simulink model "Speed_Limit_Adaptation"  (R2022b)
settings: configuration reference "CommonModelConfiguration" (kept outside this file)
undefined symbols (not defined in the file): cc_param_149, cc_param_23, cc_param_311, cc_param_36, LCFG_DSF_Timeout, LCFG_SetSpeedMinKPH_A3, LCFG_SetSpeedMinMPH_A3, LCFG_SLA_SetSpeedMaxKPH, LCFG_SLA_SetSpeedMaxMPH, LCFG_SLA_Timeout, LCFG_VehicleBrand
settings Model: Creator=RPETE142  LastModifiedBy=OTHOMSO1
settings ConfigSetRef: SourceName=CommonModelConfiguration  SourceLocation=Base Workspace

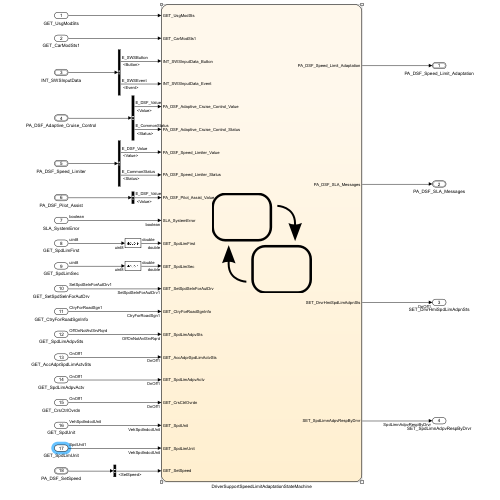
[thumbnail: Simulink's stored preview of the top-level diagram]
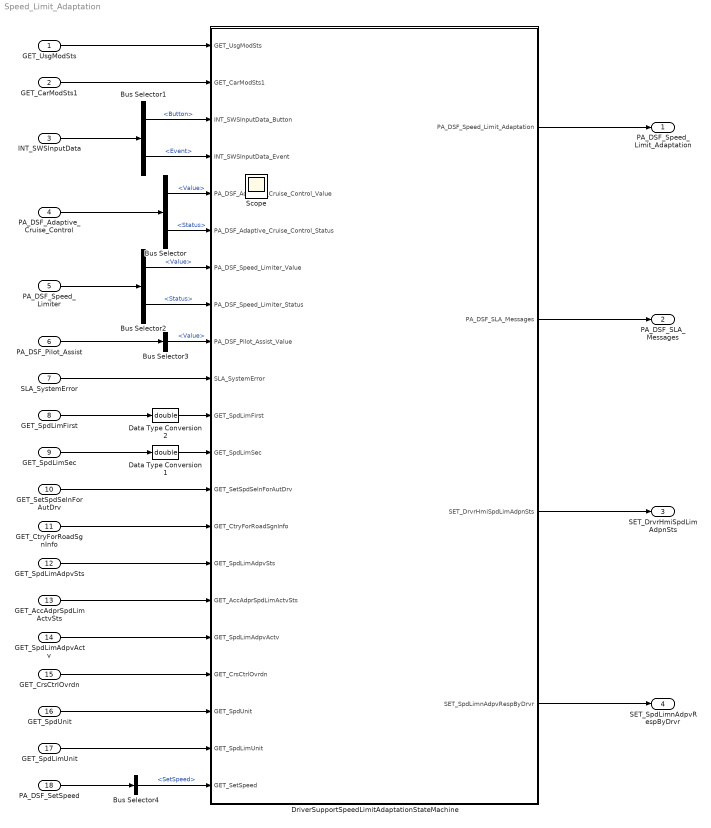
== system Speed_Limit_Adaptation ==
  GET_UsgModSts : Inport  SampleTime=0.01
  GET_CarModSts1 : Inport  Port=2
  INT_SWSInputData : Inport  Port=3  OutDataTypeStr=Bus: SWSInputData  LockScale=on
  PA_DSF_Adaptive_Cruise_Control : Inport  Port=4  OutDataTypeStr=Bus: PA_DSF_ACC
  PA_DSF_Speed_Limiter : Inport  Port=5  OutDataTypeStr=Bus: PA_DSF
  PA_DSF_Pilot_Assist : Inport  Port=6  OutDataTypeStr=Bus: PA_DSF
  SLA_SystemError : Inport  Port=7  OutDataTypeStr=boolean
  GET_SpdLimFirst : Inport  Port=8  OutDataTypeStr=SpdLimVal1
  GET_SpdLimSec : Inport  Port=9  OutDataTypeStr=SpdLimVal1
  GET_SetSpdSelnForAutDrv : Inport  Port=10  OutDataTypeStr=Enum: SetSpdSelnForAutDrv1
  GET_CtryForRoadSgnInfo : Inport  Port=11  OutDataTypeStr=Enum: CtryForRoadSgn1
  GET_SpdLimAdpvSts : Inport  Port=12  OutDataTypeStr=Enum: OffOnNotAvlSrvRqrd
  GET_AccAdprSpdLimActvSts : Inport  Port=13  OutDataTypeStr=Enum: OnOff1
  GET_SpdLimAdpvActv : Inport  Port=14  OutDataTypeStr=Enum: OnOff1
  GET_CrsCtrlOvrdn : Inport  Port=15  OutDataTypeStr=Enum: OnOff1
  GET_SpdUnit : Inport  Port=16  OutDataTypeStr=Enum: VehSpdIndcdUnit
  GET_SpdLimUnit : Inport  Port=17  OutDataTypeStr=Enum: SpdUnit1
  PA_DSF_SetSpeed : Inport  Port=18  OutDataTypeStr=Bus: PA_StatusAndValueAndDoubleAndDouble
  Bus Selector : BusSelector  OutputSignals=Value,Status
  Bus Selector1 : BusSelector  OutputSignals=Button,Event
  Bus Selector2 : BusSelector  OutputSignals=Value,Status
  Bus Selector3 : BusSelector  OutputSignals=Value
  Bus Selector4 : BusSelector  OutputSignals=SetSpeed
  Data Type Conversion1 : DataTypeConversion  OutDataTypeStr=double  SaturateOnIntegerOverflow=off  RndMeth=Floor  LockScale=on
  Data Type Conversion2 : DataTypeConversion  OutDataTypeStr=double  SaturateOnIntegerOverflow=off  RndMeth=Floor  LockScale=on
  "DriverSupportSpeedLimitAdaptationStateMachine " : Stateflow chart  TreatAsAtomicUnit=on
  PA_DSF_Speed_Limit_Adaptation : Outport  OutDataTypeStr=Bus: PA_DSF_SLA  VectorParamsAs1DForOutWhenUnconnected=off
  PA_DSF_SLA_Messages : Outport  Port=2  OutDataTypeStr=Bus: PA_DSF_Message  VectorParamsAs1DForOutWhenUnconnected=off
  SET_DrvrHmiSpdLimAdpnSts : Outport  Port=3  OutDataTypeStr=Enum: OnOff1  VectorParamsAs1DForOutWhenUnconnected=off
  SET_SpdLimnAdpvRespByDrvr : Outport  Port=4  OutDataTypeStr=Enum: SpdLimnAdpvRespByDrvr  VectorParamsAs1DForOutWhenUnconnected=off
  Scope : Scope
  wires:
  GET_UsgModSts/1 -> "DriverSupportSpeedLimitAdaptationStateMachine "/1(GET_UsgModSts)
  GET_CarModSts1/1 -> "DriverSupportSpeedLimitAdaptationStateMachine "/2(GET_CarModSts1)
  INT_SWSInputData/1 -> Bus Selector1/1
  Bus Selector1/2 -> "DriverSupportSpeedLimitAdaptationStateMachine "/4(INT_SWSInputData_Event)  "<Event>"
  Bus Selector1/1 -> "DriverSupportSpeedLimitAdaptationStateMachine "/3(INT_SWSInputData_Button)  "<Button>"
  Bus Selector/1 -> "DriverSupportSpeedLimitAdaptationStateMachine "/5(PA_DSF_Adaptive_Cruise_Control_Value)  "<Value>"
  PA_DSF_Adaptive_Cruise_Control/1 -> Bus Selector/1
  PA_DSF_Speed_Limiter/1 -> Bus Selector2/1
  PA_DSF_Pilot_Assist/1 -> Bus Selector3/1
  SLA_SystemError/1 -> "DriverSupportSpeedLimitAdaptationStateMachine "/10(SLA_SystemError)
  "DriverSupportSpeedLimitAdaptationStateMachine "/1(PA_DSF_Speed_Limit_Adaptation) -> PA_DSF_Speed_Limit_Adaptation/1
  GET_SpdLimFirst/1 -> Data Type Conversion2/1
  Data Type Conversion2/1 -> "DriverSupportSpeedLimitAdaptationStateMachine "/11(GET_SpdLimFirst)
  GET_SpdLimSec/1 -> Data Type Conversion1/1
  Data Type Conversion1/1 -> "DriverSupportSpeedLimitAdaptationStateMachine "/12(GET_SpdLimSec)
  GET_SetSpdSelnForAutDrv/1 -> "DriverSupportSpeedLimitAdaptationStateMachine "/13(GET_SetSpdSelnForAutDrv)
  GET_CtryForRoadSgnInfo/1 -> "DriverSupportSpeedLimitAdaptationStateMachine "/14(GET_CtryForRoadSgnInfo)
  Bus Selector/2 -> "DriverSupportSpeedLimitAdaptationStateMachine "/6(PA_DSF_Adaptive_Cruise_Control_Status)  "<Status>"
  Bus Selector2/1 -> "DriverSupportSpeedLimitAdaptationStateMachine "/7(PA_DSF_Speed_Limiter_Value)  "<Value>"
  Bus Selector2/2 -> "DriverSupportSpeedLimitAdaptationStateMachine "/8(PA_DSF_Speed_Limiter_Status)  "<Status>"
  Bus Selector3/1 -> "DriverSupportSpeedLimitAdaptationStateMachine "/9(PA_DSF_Pilot_Assist_Value)  "<Value>"
  "DriverSupportSpeedLimitAdaptationStateMachine "/3(SET_DrvrHmiSpdLimAdpnSts) -> SET_DrvrHmiSpdLimAdpnSts/1
  "DriverSupportSpeedLimitAdaptationStateMachine "/2(PA_DSF_SLA_Messages) -> PA_DSF_SLA_Messages/1
  GET_SpdLimAdpvSts/1 -> "DriverSupportSpeedLimitAdaptationStateMachine "/15(GET_SpdLimAdpvSts)
  GET_AccAdprSpdLimActvSts/1 -> "DriverSupportSpeedLimitAdaptationStateMachine "/16(GET_AccAdprSpdLimActvSts)
  GET_SpdLimAdpvActv/1 -> "DriverSupportSpeedLimitAdaptationStateMachine "/17(GET_SpdLimAdpvActv)
  "DriverSupportSpeedLimitAdaptationStateMachine "/4(SET_SpdLimnAdpvRespByDrvr) -> SET_SpdLimnAdpvRespByDrvr/1
  GET_CrsCtrlOvrdn/1 -> "DriverSupportSpeedLimitAdaptationStateMachine "/18(GET_CrsCtrlOvrdn)
  GET_SpdUnit/1 -> "DriverSupportSpeedLimitAdaptationStateMachine "/19(GET_SpdUnit)
  PA_DSF_SetSpeed/1 -> Bus Selector4/1
  Bus Selector4/1 -> "DriverSupportSpeedLimitAdaptationStateMachine "/21(GET_SetSpeed)  "<SetSpeed>"
  GET_SpdLimUnit/1 -> "DriverSupportSpeedLimitAdaptationStateMachine "/20(GET_SpdLimUnit)

== stateflow chart Speed_Limit_Adaptation/DriverSupportSpeedLimitAdaptationStateMachine  ==
  state CARCONFIG_INVALID
    entry:
    PA_DSF_Speed_Limit_Adaptation.Status = E_CommonStatus.NotPresent;
    PA_DSF_Speed_Limit_Adaptation.Value = E_DSF_Value.DSF_Off;
    PA_DSF_Speed_Limit_Adaptation.Format = false;
    PA_DSF_Speed_Limit_Adaptation.Data = 0;
    PA_DSF_SLA_Messages.Status = E_CommonStatus.NotPresent;
    PA_DSF_SLA_Messages.Value = E_DSF_Messages.Messages_Off;
    SET_DrvrHmiSpdLimAdpnSts = OnOff1.OnOff1_Off;
  state SYSTEM_OK
    state isActive = activationCheck [function]
      (default) -> (junction 35)
      (junction 28) -> (junction 1896) [order 1] : [PA_DSF_Speed_Limiter_Status==E_CommonStatus.Available &&...
          | cc_param_36 > 2]
      (junction 35) -> (junction 28) [order 1] : [GET_UsgModSts==UsgModSts1.UsgModSts1_UsgModDrvg &&...
          | GET_CarModSts1==CarModSts1.CarModSts1_CarModNorm]
      (junction 35) -> (junction 31) [order 2] : {isActive = false;}
      (junction 28) -> (junction 1894) [order 2]
      (junction 1896) -> (junction 1898)
      (junction 1894) -> (junction 1898) [order 1] : [PA_DSF_Adaptive_Cruise_Control_Status==E_CommonStatus.Available &&...
          | (cc_param_23 > 2 && mod(cc_param_149,2)==1) &&...
          | (cc_param_149~=1)]
      (junction 1894) -> (junction 4418) [order 2]
      (junction 1898) -> (junction 4414)
      (junction 4414) -> (junction 4418) [order 2]
      (junction 4418) -> (junction 4382) : {isActive = false;}
      (junction 4414) -> (junction 30) [order 1] : [(GET_AccAdprSpdLimActvSts==OnOff1.OnOff1_On &&...
          | LCFG_VehicleBrand==1) || LCFG_VehicleBrand==2]
          | {isActive = true;}
      (junction 30) -> (junction 4382)
      (junction 4382) -> (junction 31)
      (junction 31) -> (junction 4386)
    state NOT_ACTIVE
      entry:
      PA_DSF_Speed_Limit_Adaptation.Status = E_CommonStatus.Disabled;
      PA_DSF_Speed_Limit_Adaptation.Data = 0;
      PA_DSF_SLA_Messages.Status = E_CommonStatus.Disabled;
      PA_DSF_SLA_Messages.Value = E_DSF_Messages.Messages_Off;
      SET_DrvrHmiSpdLimAdpnSts = OnOff1.OnOff1_Off;
      PA_DSF_SLA_Messages.Value = E_DSF_Messages.Messages_Off;
      PA_DSF_Speed_Limit_Adaptation.Value = E_DSF_Value.DSF_Off;
    state ACTIVE
      entry:
      PA_DSF_SLA_Messages.Status = E_CommonStatus.Disabled;
      PA_DSF_SLA_Messages.Value = E_DSF_Messages.Messages_Off;
      PA_DSF_Speed_Limit_Adaptation.Status = E_CommonStatus.Available;
      state DATA [parallel]
        settings: executionOrder=1
        state retVal = isSpdLimSec [function]
          (default) -> (junction 3783)
          (junction 3783) -> (junction 3784) [order 1] : [GET_SetSpdSelnForAutDrv==SetSpdSelnForAutDrv1.SetSpdSelnForAutDrv1_AdjSetSpdToCmngSpdLim &&...
              | PA_DSF_Adaptive_Cruise_Control_Status==E_CommonStatus.Available]
          (junction 3783) -> (junction 3786) [order 2] : {retVal = false;}
          (junction 3784) -> (junction 3787) : {retVal = true;}
          (junction 3787) -> (junction 3786)
          (junction 3786) -> (junction 3789)
        state spd = SLA_Speed(SpdLim) [function]
          (default) -> (junction 4560)
          (junction 4560) -> (junction 4558) [order 1] : %Convert to SpdUnit for Argus3
              | [SpdLim>0 && SpdLim<254 && cc_param_311==3 &&...
              | ((GET_SpdLimUnit==SpdUnit1.SpdUnit1_KiloMtrPerHr &&...
              | GET_SpdUnit==VehSpdIndcdUnit.VehSpdIndcdUnit_Mph) ||...
              | (GET_SpdLimUnit==SpdUnit1.SpdUnit1_MilePerHr &&...
              | GET_SpdUnit==VehSpdIndcdUnit.VehSpdIndcdUnit_Kmph))]
          (junction 4560) -> (junction 4555) [order 2]
          (junction 4558) -> (junction 4563)
          (junction 4563) -> (junction 4561) [order 1] : [GET_SpdLimUnit==SpdUnit1.SpdUnit1_KiloMtrPerHr]
          (junction 4563) -> (junction 4559) [order 2] : {SpdLim = 103/64*SpdLim;}
          (junction 4561) -> (junction 4562) : {SpdLim = 64/103*SpdLim;}
          (junction 4559) -> (junction 4555) : %Round down to nearest integer
              | {SpdLim = floor(SpdLim);}
          (junction 4562) -> (junction 4559)
          (junction 4555) -> (junction 4473)
          (junction 4473) -> (junction 4474) [order 1] : %Free speed
              | [SpdLim==254]
          (junction 4474) -> (junction 4527) [order 1] : [GET_SpdUnit==VehSpdIndcdUnit.VehSpdIndcdUnit_Mph]
          (junction 4473) -> (junction 4475) [order 2] : {spd = SpdLim;}
          (junction 4474) -> (junction 4476) [order 2] : {spd = max(LCFG_SLA_SetSpeedMaxKPH, GET_SetSpeed);}
          (junction 4527) -> (junction 4529) : {spd = max(LCFG_SLA_SetSpeedMaxMPH, GET_SetSpeed);}
          (junction 4476) -> (junction 4475)
          (junction 4529) -> (junction 4476)
          (junction 4475) -> (junction 4477)
        state SPD_LIM_FIRST
          entry, during:
          PA_DSF_Speed_Limit_Adaptation.Data = SLA_Speed(GET_SpdLimFirst);
        state SPD_LIM_SEC
          entry, during:
          PA_DSF_Speed_Limit_Adaptation.Data = SLA_Speed(GET_SpdLimSec);
        (default) -> (junction 3807)
        (junction 3807) -> SPD_LIM_FIRST [order 2]
        (junction 3807) -> (junction 3810) [order 1] : [isSpdLimSec()]
        SPD_LIM_SEC -> SPD_LIM_FIRST : [~isSpdLimSec()]
        SPD_LIM_FIRST -> SPD_LIM_SEC : [isSpdLimSec()]
        (junction 3810) -> SPD_LIM_SEC
      state SPEED_LIMIT_ADAPTATION [parallel]
        entry:
        PA_DSF_Speed_Limit_Adaptation.Status = E_CommonStatus.Available;
        settings: executionOrder=2
        state retVal = cruiseActive [function]
          (default) -> (junction 4304)
          (junction 4304) -> (junction 4305) [order 1] : [PA_DSF_Speed_Limiter_Status==E_CommonStatus.Available ]
          (junction 4305) -> (junction 4306) [order 2]
          (junction 4305) -> (junction 4309) [order 1] : [PA_DSF_Speed_Limiter_Value==E_DSF_Value.DSF_Active]
          (junction 4306) -> (junction 4314) : {retVal = false;}
          (junction 4304) -> (junction 4307) [order 2]
          (junction 4307) -> (junction 4308) [order 1] : [PA_DSF_Adaptive_Cruise_Control_Status==E_CommonStatus.Available ]
          (junction 4308) -> (junction 4309) [order 1] : [PA_DSF_Adaptive_Cruise_Control_Value==E_DSF_Value.DSF_Active ||...
              | PA_DSF_Adaptive_Cruise_Control_Value==E_DSF_Value.DSF_StopMode]
          (junction 4307) -> (junction 4310) [order 2]
          (junction 4308) -> (junction 4311) [order 2]
          (junction 4309) -> (junction 4313) : {retVal = true;}
          (junction 4310) -> (junction 4311)
          (junction 4311) -> (junction 4312) : {retVal = false;}
          (junction 4313) -> (junction 4312)
          (junction 4314) -> (junction 4313)
          (junction 4312) -> (junction 4315)
        state retVal = cruiseActivation [function]
          (default) -> (junction 4336)
          (junction 4336) -> (junction 4334) [order 1] : [PA_DSF_Speed_Limiter_Status==E_CommonStatus.Available ]
          (junction 4334) -> (junction 4335) [order 2]
          (junction 4336) -> (junction 4339) [order 2]
          (junction 4334) -> (junction 4337) [order 1] : [hasChangedTo(PA_DSF_Speed_Limiter_Value,E_DSF_Value.DSF_Active)]
          (junction 4335) -> (junction 4344) : {retVal = false;}
          (junction 4339) -> (junction 4338) [order 1] : [PA_DSF_Adaptive_Cruise_Control_Status==E_CommonStatus.Available ]
          (junction 4338) -> (junction 4337) [order 1] : [hasChangedTo(PA_DSF_Adaptive_Cruise_Control_Value,E_DSF_Value.DSF_Active) ||...
              | hasChangedTo(PA_DSF_Adaptive_Cruise_Control_Value,E_DSF_Value.DSF_StopMode)]
          (junction 4339) -> (junction 4341) [order 2]
          (junction 4338) -> (junction 4340) [order 2]
          (junction 4337) -> (junction 4343) : {retVal = true;}
          (junction 4341) -> (junction 4340)
          (junction 4340) -> (junction 4342) : {retVal = false;}
          (junction 4343) -> (junction 4342)
          (junction 4344) -> (junction 4343)
          (junction 4342) -> (junction 4345)
        state POLESTAR
          state HIDDEN
            entry:
            PA_DSF_Speed_Limit_Adaptation.Value=E_DSF_Value.DSF_Off;
          state DISPLAYED
            entry: SET_DrvrHmiSpdLimAdpnSts = OnOff1.OnOff1_On;
            state NOT_SELECTED
              entry:
              PA_DSF_Speed_Limit_Adaptation.Value=E_DSF_Value.DSF_Not_Selected;
              isVisible = true;
            state SELECTED
              entry:
              SET_DrvrHmiSpdLimAdpnSts = OnOff1.OnOff1_On;
              state OFF
                entry:
                PA_DSF_Speed_Limit_Adaptation.Value=E_DSF_Value.DSF_Selected;
              state ON
                entry:
                state STANDBY
                  entry:
                  PA_DSF_Speed_Limit_Adaptation.Value=E_DSF_Value.DSF_Standby
                state ACTIVE
                  entry:
                  PA_DSF_Speed_Limit_Adaptation.Value=E_DSF_Value.DSF_Active;
                (default) -> (junction 4164)
                (junction 4164) -> (junction 4159) [order 1] : [PA_DSF_Adaptive_Cruise_Control_Status ~= E_CommonStatus.Available ||...
                    | (GET_SpdLimAdpvSts == OffOnNotAvlSrvRqrd.OffOnNotAvlSrvRqrd_On &&...
                    | GET_SetSpdSelnForAutDrv~=SetSpdSelnForAutDrv1.SetSpdSelnForAutDrv1_KeepSetSpdValPrsnt) ]
                (junction 4164) -> (junction 4167) [order 2]
                (junction 4159) -> SYSTEM_OK.ACTIVE.SPEED_LIMIT_ADAPTATION.POLESTAR.DISPLAYED.SELECTED.ON.ACTIVE
                (junction 4167) -> SYSTEM_OK.ACTIVE.SPEED_LIMIT_ADAPTATION.POLESTAR.DISPLAYED.SELECTED.ON.STANDBY
                SYSTEM_OK.ACTIVE.SPEED_LIMIT_ADAPTATION.POLESTAR.DISPLAYED.SELECTED.ON.STANDBY -> SYSTEM_OK.ACTIVE.SPEED_LIMIT_ADAPTATION.POLESTAR.DISPLAYED.SELECTED.ON.ACTIVE : [(GET_SpdLimAdpvSts == OffOnNotAvlSrvRqrd.OffOnNotAvlSrvRqrd_On &&...
                    | GET_SetSpdSelnForAutDrv~=SetSpdSelnForAutDrv1.SetSpdSelnForAutDrv1_KeepSetSpdValPrsnt) ]
                SYSTEM_OK.ACTIVE.SPEED_LIMIT_ADAPTATION.POLESTAR.DISPLAYED.SELECTED.ON.ACTIVE -> SYSTEM_OK.ACTIVE.SPEED_LIMIT_ADAPTATION.POLESTAR.DISPLAYED.SELECTED.ON.STANDBY : [PA_DSF_Adaptive_Cruise_Control_Status == E_CommonStatus.Available &&...
                    | (GET_SpdLimAdpvSts ~= OffOnNotAvlSrvRqrd.OffOnNotAvlSrvRqrd_On ||...
                    | GET_SetSpdSelnForAutDrv==SetSpdSelnForAutDrv1.SetSpdSelnForAutDrv1_KeepSetSpdValPrsnt)]
              (default) -> (junction 3922)
              (junction 3922) -> (junction 3921) [order 1] : [cruiseActive()]
              (junction 3921) -> ON
              (junction 3922) -> SYSTEM_OK.ACTIVE.SPEED_LIMIT_ADAPTATION.POLESTAR.DISPLAYED.SELECTED.OFF [order 2]
              SYSTEM_OK.ACTIVE.SPEED_LIMIT_ADAPTATION.POLESTAR.DISPLAYED.SELECTED.OFF -> ON : [cruiseActivation()]
              ON -> SYSTEM_OK.ACTIVE.SPEED_LIMIT_ADAPTATION.POLESTAR.DISPLAYED.SELECTED.OFF : [~cruiseActive()]
            (default) -> NOT_SELECTED
            NOT_SELECTED -> SELECTED : [INT_SWSInputData_Button == E_SWSButton.BtnL2Req &&...
                | hasChangedTo(INT_SWSInputData_Event, E_SWSEvent.Push)]
            SELECTED -> NOT_SELECTED : [INT_SWSInputData_Button == E_SWSButton.BtnL2Req &&...
                | hasChangedTo(INT_SWSInputData_Event, E_SWSEvent.Push)]
          (default) -> (junction 3905)
          (junction 3905) -> HIDDEN [order 1] : [isVisible == false && PA_DSF_Pilot_Assist_Value == E_DSF_Value.DSF_Off]
          (junction 3905) -> DISPLAYED [order 2]
          HIDDEN -> DISPLAYED [order 2] : [cruiseActive() || (PA_DSF_Pilot_Assist_Value == E_DSF_Value.DSF_Selected)]
          HIDDEN -> SELECTED [order 1] : [INT_SWSInputData_Button == E_SWSButton.BtnL2Req &&...
              | hasChangedTo(INT_SWSInputData_Event, E_SWSEvent.Push)]
        state VOLVO
          state ON_A3
            state isValid = valid_spd [function]
              (default) -> (junction 4487)
              (junction 4487) -> (junction 4488) [order 1] : [GET_SpdUnit==VehSpdIndcdUnit.VehSpdIndcdUnit_Mph]
              (junction 4488) -> (junction 4519) [order 2]
              (junction 4487) -> (junction 4513) [order 2]
              (junction 4488) -> (junction 4511) [order 1] : %Outside SLA speed limits (mph) or no change
                  | [PA_DSF_Speed_Limit_Adaptation.Data<LCFG_SetSpeedMinMPH_A3 ||...
                  | PA_DSF_Speed_Limit_Adaptation.Data>LCFG_SLA_SetSpeedMaxMPH ||...
                  | PA_DSF_Speed_Limit_Adaptation.Data==GET_SetSpeed]
              (junction 4519) -> (junction 4521)
              (junction 4513) -> (junction 4511) [order 1] : %Outside SLA speed limits (kph) or no change
                  | [PA_DSF_Speed_Limit_Adaptation.Data<LCFG_SetSpeedMinKPH_A3 ||...
                  | PA_DSF_Speed_Limit_Adaptation.Data>LCFG_SLA_SetSpeedMaxKPH ||...
                  | PA_DSF_Speed_Limit_Adaptation.Data==GET_SetSpeed]
              (junction 4513) -> (junction 4516) [order 2]
              (junction 4511) -> (junction 4490) : {isValid = false}
              (junction 4521) -> (junction 4516)
              (junction 4516) -> (junction 4489) : {isValid = true}
              (junction 4490) -> (junction 4489)
              (junction 4489) -> (junction 4491)
            state isRejected = checkRejection [function]
              (default) -> (junction 4435)
              (junction 4435) -> (junction 4437) [order 1] : %Up/down button pressed or accelerator pedal at set speed decrease
                  | [(INT_SWSInputData_Button==E_SWSButton.BtnL4Req ||...
                  | INT_SWSInputData_Button==E_SWSButton.BtnL5Req) &&...
                  | INT_SWSInputData_Event==E_SWSEvent.Release ||...
                  | (GET_SetSpdSelnForAutDrv==...
                  | SetSpdSelnForAutDrv1.SetSpdSelnForAutDrv1_AdjSetSpdToCmngSpdLim &&...
                  | GET_CrsCtrlOvrdn==OnOff1.OnOff1_On)]
              (junction 4435) -> (junction 4441) [order 2] : {isRejected = false}
              (junction 4437) -> (junction 4439) : {isRejected = true}
              (junction 4439) -> (junction 4441)
              (junction 4441) -> (junction 4444)
            state STANDBY
              entry:
              PA_DSF_Speed_Limit_Adaptation.Value = E_DSF_Value.DSF_Standby;
              SET_SpdLimnAdpvRespByDrvr = SpdLimnAdpvRespByDrvr.NoResponse;
            state ACTIVE
              entry:
              PA_DSF_Speed_Limit_Adaptation.Value = E_DSF_Value.DSF_Active;
            state REJECTED
              entry:
              SET_SpdLimnAdpvRespByDrvr = SpdLimnAdpvRespByDrvr.Rejected;
              PA_DSF_Speed_Limit_Adaptation.Value = E_DSF_Value.DSF_Overridden;
            (default) -> (junction 4401)
            (junction 4401) -> (junction 4402) [order 1] : [GET_SpdLimAdpvSts==OffOnNotAvlSrvRqrd.OffOnNotAvlSrvRqrd_On &&...
                | GET_SpdLimAdpvActv==OnOff1.OnOff1_On &&...
                | valid_spd && GET_SetSpdSelnForAutDrv~=...
                | SetSpdSelnForAutDrv1.SetSpdSelnForAutDrv1_KeepSetSpdValPrsnt]
            (junction 4401) -> SYSTEM_OK.ACTIVE.SPEED_LIMIT_ADAPTATION.VOLVO.ON_A3.STANDBY [order 2]
            (junction 4402) -> SYSTEM_OK.ACTIVE.SPEED_LIMIT_ADAPTATION.VOLVO.ON_A3.ACTIVE
            SYSTEM_OK.ACTIVE.SPEED_LIMIT_ADAPTATION.VOLVO.ON_A3.STANDBY -> SYSTEM_OK.ACTIVE.SPEED_LIMIT_ADAPTATION.VOLVO.ON_A3.ACTIVE : [(GET_SpdLimAdpvSts==OffOnNotAvlSrvRqrd.OffOnNotAvlSrvRqrd_On &&...
                | hasChangedTo(GET_SpdLimAdpvActv, OnOff1.OnOff1_On) &&...
                | valid_spd && GET_SetSpdSelnForAutDrv~=...
                | SetSpdSelnForAutDrv1.SetSpdSelnForAutDrv1_KeepSetSpdValPrsnt)]
            SYSTEM_OK.ACTIVE.SPEED_LIMIT_ADAPTATION.VOLVO.ON_A3.ACTIVE -> SYSTEM_OK.ACTIVE.SPEED_LIMIT_ADAPTATION.VOLVO.ON_A3.STANDBY [order 1] : %No rejection for SL
                | [PA_DSF_Speed_Limiter_Status==E_CommonStatus.Available]
            SYSTEM_OK.ACTIVE.SPEED_LIMIT_ADAPTATION.VOLVO.ON_A3.ACTIVE -> SYSTEM_OK.ACTIVE.SPEED_LIMIT_ADAPTATION.VOLVO.ON_A3.STANDBY [order 3] : [(GET_SpdLimAdpvSts~=OffOnNotAvlSrvRqrd.OffOnNotAvlSrvRqrd_On ||...
                | GET_SetSpdSelnForAutDrv==...
                | SetSpdSelnForAutDrv1.SetSpdSelnForAutDrv1_KeepSetSpdValPrsnt) ||...
                | after(LCFG_SLA_Timeout, sec)]
            SYSTEM_OK.ACTIVE.SPEED_LIMIT_ADAPTATION.VOLVO.ON_A3.ACTIVE -> REJECTED [order 2] : [checkRejection]
            REJECTED -> SYSTEM_OK.ACTIVE.SPEED_LIMIT_ADAPTATION.VOLVO.ON_A3.STANDBY : [after(LCFG_SLA_Timeout, sec)]
          state OFF
            entry:
            PA_DSF_Speed_Limit_Adaptation.Value = E_DSF_Value.DSF_Selected;
          state ON_A2
            entry:
            SET_SpdLimnAdpvRespByDrvr = SpdLimnAdpvRespByDrvr.NoResponse;
            state STANDBY
              entry:
              PA_DSF_Speed_Limit_Adaptation.Value =...
              E_DSF_Value.DSF_Standby;
            state ACTIVE
              entry:
              PA_DSF_Speed_Limit_Adaptation.Value =...
              E_DSF_Value.DSF_Active;
            (default) -> (junction 4451)
            (junction 4451) -> (junction 4452) [order 1] : [PA_DSF_Adaptive_Cruise_Control_Status ~= E_CommonStatus.Available ||...
                | (GET_SpdLimAdpvSts == OffOnNotAvlSrvRqrd.OffOnNotAvlSrvRqrd_On &&...
                | GET_SetSpdSelnForAutDrv~=SetSpdSelnForAutDrv1.SetSpdSelnForAutDrv1_KeepSetSpdValPrsnt) ]
            (junction 4451) -> SYSTEM_OK.ACTIVE.SPEED_LIMIT_ADAPTATION.VOLVO.ON_A2.STANDBY [order 2]
            (junction 4452) -> SYSTEM_OK.ACTIVE.SPEED_LIMIT_ADAPTATION.VOLVO.ON_A2.ACTIVE
            SYSTEM_OK.ACTIVE.SPEED_LIMIT_ADAPTATION.VOLVO.ON_A2.STANDBY -> SYSTEM_OK.ACTIVE.SPEED_LIMIT_ADAPTATION.VOLVO.ON_A2.ACTIVE : [(GET_SpdLimAdpvSts==OffOnNotAvlSrvRqrd.OffOnNotAvlSrvRqrd_On &&...
                | GET_SetSpdSelnForAutDrv~=SetSpdSelnForAutDrv1.SetSpdSelnForAutDrv1_KeepSetSpdValPrsnt) ]
            SYSTEM_OK.ACTIVE.SPEED_LIMIT_ADAPTATION.VOLVO.ON_A2.ACTIVE -> SYSTEM_OK.ACTIVE.SPEED_LIMIT_ADAPTATION.VOLVO.ON_A2.STANDBY : [PA_DSF_Adaptive_Cruise_Control_Status==E_CommonStatus.Available &&...
                | (GET_SpdLimAdpvSts~=OffOnNotAvlSrvRqrd.OffOnNotAvlSrvRqrd_On ||...
                | GET_SetSpdSelnForAutDrv==SetSpdSelnForAutDrv1.SetSpdSelnForAutDrv1_KeepSetSpdValPrsnt)]
          (default) -> (junction 4412)
          (junction 4412) -> (junction 4466) [order 1] : [cruiseActive()]
          (junction 4466) -> ON_A2 [order 2] : %Not Argus3
          (junction 4466) -> ON_A3 [order 1] : %Argus3
              | [cc_param_311==3]
          (junction 4412) -> SYSTEM_OK.ACTIVE.SPEED_LIMIT_ADAPTATION.VOLVO.OFF [order 2]
          ON_A3 -> SYSTEM_OK.ACTIVE.SPEED_LIMIT_ADAPTATION.VOLVO.OFF : [~cruiseActive()]
          SYSTEM_OK.ACTIVE.SPEED_LIMIT_ADAPTATION.VOLVO.OFF -> (junction 4463) : [cruiseActivation()]
          (junction 4463) -> ON_A3 [order 1] : %Argus3
              | [cc_param_311==3]
          (junction 4463) -> ON_A2 [order 2] : %Not Argus3
          ON_A2 -> SYSTEM_OK.ACTIVE.SPEED_LIMIT_ADAPTATION.VOLVO.OFF : [~cruiseActive()]
        (default) -> (junction 4390)
        (junction 4390) -> VOLVO [order 2]
        (junction 4390) -> POLESTAR [order 1] : [LCFG_VehicleBrand==2]
      state FORMAT [parallel]
        settings: executionOrder=3
        state retVal = isUSAorCanada [function]
          (default) -> (junction 4214)
          (junction 4214) -> (junction 4215) [order 1] : [GET_CtryForRoadSgnInfo== CtryForRoadSgn1.CtryForRoadSgn1_USA ...
              | || GET_CtryForRoadSgnInfo== CtryForRoadSgn1.CtryForRoadSgn1_Canada]
          (junction 4214) -> (junction 4216) [order 2] : {retVal = false;}
          (junction 4215) -> (junction 4217) : {retVal = true;}
          (junction 4217) -> (junction 4216)
          (junction 4216) -> (junction 4218)
        state REST_OF_WORLD
          entry:
          PA_DSF_Speed_Limit_Adaptation.Format = false;
        state USA_OR_CANADA
          entry:
          PA_DSF_Speed_Limit_Adaptation.Format = true;
        (junction 4202) -> REST_OF_WORLD
        (junction 4203) -> (junction 4202) [order 2]
        REST_OF_WORLD -> USA_OR_CANADA : [isUSAorCanada()]
        USA_OR_CANADA -> REST_OF_WORLD : [~isUSAorCanada()]
        (default) -> (junction 4203)
        (junction 4203) -> (junction 4204) [order 1] : [isUSAorCanada()]
        (junction 4204) -> USA_OR_CANADA
    (default) -> (junction 4363)
    (junction 4363) -> NOT_ACTIVE [order 1] : [~activationCheck()]
    (junction 4363) -> (junction 4365) [order 2]
    NOT_ACTIVE -> SYSTEM_OK.ACTIVE : [activationCheck()]
    SYSTEM_OK.ACTIVE -> NOT_ACTIVE : [~activationCheck()]
    (junction 4365) -> SYSTEM_OK.ACTIVE
  state SYSTEM_ERROR
    entry:
    PA_DSF_Speed_Limit_Adaptation.Status=E_CommonStatus.SystemError;
    PA_DSF_Speed_Limit_Adaptation.Data = 0;
    PA_DSF_SLA_Messages.Status = E_CommonStatus.SystemError;
    PA_DSF_SLA_Messages.Value = E_DSF_Messages.Messages_Off;
    SET_DrvrHmiSpdLimAdpnSts = OnOff1.OnOff1_Off;
    state retVal = slaActivationReq [function]
      (default) -> (junction 4179)
      (junction 4179) -> (junction 4180) [order 1] : [INT_SWSInputData_Button == E_SWSButton.BtnL2Req ...
          | && hasChangedTo(INT_SWSInputData_Event, E_SWSEvent.Push)...
          | && PA_DSF_Adaptive_Cruise_Control_Status == E_CommonStatus.Available ]
      (junction 4179) -> (junction 4181) [order 2] : {retVal=false;}
      (junction 4180) -> (junction 4182) : {retVal=true;}
      (junction 4182) -> (junction 4181)
      (junction 4181) -> (junction 4183)
    state CANCEL_WARNING
      entry:
      PA_DSF_SLA_Messages.Value=E_DSF_Messages.Messages_CancelWarning;
      PA_DSF_Speed_Limit_Adaptation.Value=E_DSF_Value.DSF_Off;
    state UNAVAILABLE
      entry:
      PA_DSF_SLA_Messages.Value=E_DSF_Messages.Messages_Unavailable;
    state NO_MESSAGES
      entry:
      PA_DSF_SLA_Messages.Value=E_DSF_Messages.Messages_Off;
      PA_DSF_Speed_Limit_Adaptation.Value=E_DSF_Value.DSF_Off;
    (default) -> (junction 4175)
    (junction 4175) -> (junction 4176) [order 1] : [ PA_DSF_Speed_Limit_Adaptation.Value == E_DSF_Value.DSF_Active ||...
        | PA_DSF_Speed_Limit_Adaptation.Value == E_DSF_Value.DSF_Standby]
    (junction 4175) -> NO_MESSAGES [order 2]
    (junction 4176) -> CANCEL_WARNING
    UNAVAILABLE -> UNAVAILABLE [order 2] : [slaActivationReq()]
    CANCEL_WARNING -> UNAVAILABLE [order 2] : [slaActivationReq()]
    UNAVAILABLE -> NO_MESSAGES [order 1] : [after(LCFG_DSF_Timeout, sec)]
    NO_MESSAGES -> UNAVAILABLE : [slaActivationReq()]
    CANCEL_WARNING -> NO_MESSAGES [order 1] : [after(LCFG_DSF_Timeout, sec)]
  (default) -> (junction 284)
  (junction 284) -> CARCONFIG_INVALID [order 2]
  (junction 284) -> (junction 287) [order 1] : [(cc_param_23>2 && mod(cc_param_149,2)==1 &&...
      | cc_param_149~=1) || cc_param_36>2 && cc_param_149>1]
  (junction 287) -> SYSTEM_OK [order 2]
  (junction 287) -> (junction 3761) [order 1] : [SLA_SystemError==true ||...
      | INT_SWSInputData_Event==E_SWSEvent.ButtonStuck ||...
      | GET_SpdLimAdpvSts==...
      | OffOnNotAvlSrvRqrd.OffOnNotAvlSrvRqrd_SrvRqrd]
  SYSTEM_OK -> SYSTEM_ERROR : [SLA_SystemError==true ||...
      |  INT_SWSInputData_Event==E_SWSEvent.ButtonStuck ||...
      | GET_SpdLimAdpvSts==...
      | OffOnNotAvlSrvRqrd.OffOnNotAvlSrvRqrd_SrvRqrd]
  SYSTEM_ERROR -> SYSTEM_OK : [SLA_SystemError==false &&...
      |  INT_SWSInputData_Event~=E_SWSEvent.ButtonStuck &&...
      | GET_SpdLimAdpvSts~=...
      | OffOnNotAvlSrvRqrd.OffOnNotAvlSrvRqrd_SrvRqrd]
  (junction 3761) -> SYSTEM_ERROR
  data: isActive function_output; retVal function_output; SpdLim function_input; spd function_output; retVal function_output; retVal function_output; isValid function_output; isRejected function_output; retVal function_output; retVal function_output; GET_UsgModSts input Enum: UsgModSts1; GET_CarModSts1 input Enum: CarModSts1; INT_SWSInputData_Button input Enum: E_SWSButton; INT_SWSInputData_Event input Enum: E_SWSEvent; PA_DSF_Speed_Limit_Adaptation output Bus: PA_DSF_SLA =0; PA_DSF_SLA_Messages output Bus: PA_DSF_Message =0; PA_DSF_Adaptive_Cruise_Control_Value input Enum: E_DSF_Value; PA_DSF_Adaptive_Cruise_Control_Status input Enum: E_CommonStatus; PA_DSF_Speed_Limiter_Value input Enum: E_DSF_Value; PA_DSF_Speed_Limiter_Status input Enum: E_CommonStatus; cc_param_23 parameter double; cc_param_149 parameter double; cc_param_36 parameter double; PA_DSF_Pilot_Assist_Value input Enum: E_DSF_Value; SLA_SystemError input boolean; GET_SpdLimFirst input double; GET_SpdLimSec input double; GET_SetSpdSelnForAutDrv input Enum: SetSpdSelnForAutDrv1; isVisible local boolean =false; GET_CtryForRoadSgnInfo input Enum: CtryForRoadSgn1; SET_DrvrHmiSpdLimAdpnSts output Enum: OnOff1; GET_SpdLimAdpvSts input Enum: OffOnNotAvlSrvRqrd; LCFG_DSF_Timeout parameter; LCFG_VehicleBrand parameter single; GET_AccAdprSpdLimActvSts input Enum: OnOff1; GET_SpdLimAdpvActv input; SET_SpdLimnAdpvRespByDrvr output; GET_CrsCtrlOvrdn input; LCFG_SLA_Timeout parameter; cc_param_311 parameter; GET_SpdUnit input Enum: VehSpdIndcdUnit; GET_SpdLimUnit input; GET_SetSpeed input double; LCFG_SLA_SetSpeedMaxMPH parameter; LCFG_SLA_SetSpeedMaxKPH parameter; LCFG_SetSpeedMinKPH_A3 parameter; LCFG_SetSpeedMinMPH_A3 parameter
